simulink model "newsinglecapacitor"  (R2022a)
settings: Solver=VariableStepAuto  StartTime=0.0  StopTime=inf  RelTol=1e-3
undefined symbols (not defined in the file): Ion, Lithium
libraries: spsIdealSwitchLib x9, spsBatteryLib x4, spsCurrentMeasurementLib x1, simulink x1, spsSeriesRLCBranchLib x1, spsVoltageMeasurementLib x1, spspowerguiLib x1
settings Model: Creator=mluser  LastModifiedBy=LENOVO

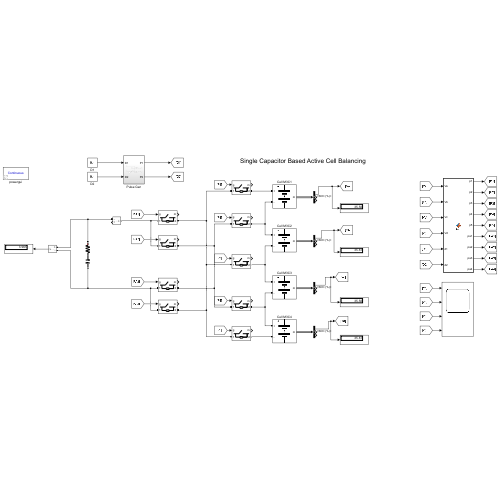
[thumbnail: Simulink's stored preview of the top-level diagram]
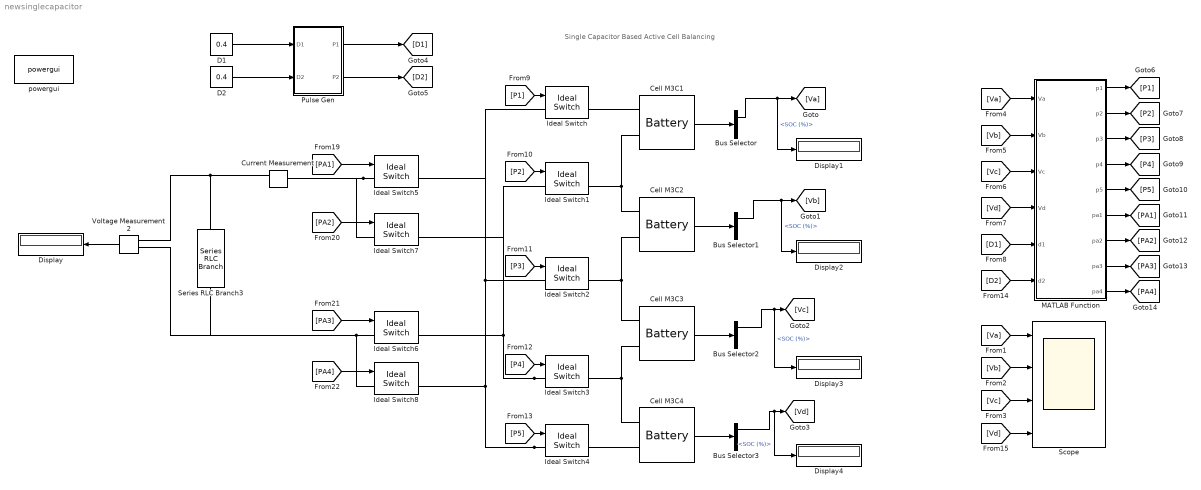
== system newsinglecapacitor ==
  note: Single Capacitor Based Active Cell Balancing
  Bus Selector{,1..3} (4 alike) : BusSelector  OutputSignals=SOC (%),Voltage (V),Current (A)
  Cell M3C1 : spsBatteryLib/Battery  BatType=Lithium-Ion  ShowTempParam=off  ThermalPreset=no  ShowAgeParam=off  NomV=3.7  NomQ=2.6  SOC=35  Batt_Tr=30  PresetModel=off  MaxQ=2.6  MinV=2.775  FullV=4.3068  Dis_rate=1.1304  R=0.014231  Normal_OP=2.3513  expZone="[3.9974      0.12774]"  current=[6.5 13 32.5]  Units=Time  Tci=20  NomT=20  T2=-30  MaxQ2=4.8  FullV2=7.1  Normal_OP2=5.655  expZone2="[6.58           1]"  Rca=0.6  ti=2000  Dp=0  Neq0=0  Tsim=1e6  Ta1=25  Qeol=5.4*0.9  Reol=0.013333*1.2  Char_age=[2.3478, 3]  Dis_age=[2.3478, 10]  N1=1500  N2=10500  N3=1000  N4=1400  Ta2=45  N5=950
  Cell M3C2 : spsBatteryLib/Battery  BatType=Lithium-Ion  ShowTempParam=off  ThermalPreset=no  ShowAgeParam=off  NomV=3.7  NomQ=2.6  SOC=37  Batt_Tr=30  PresetModel=off  MaxQ=2.6  MinV=2.775  FullV=4.3068  Dis_rate=1.1304  R=0.014231  Normal_OP=2.3513  expZone="[3.9974      0.12774]"  current=[6.5 13 32.5]  Units=Time  Tci=20  NomT=20  T2=-30  MaxQ2=4.8  FullV2=7.1  Normal_OP2=5.655  expZone2="[6.58           1]"  Rca=0.6  ti=2000  Dp=0  Neq0=0  Tsim=1e6  Ta1=25  Qeol=5.4*0.9  Reol=0.013333*1.2  Char_age=[2.3478, 3]  Dis_age=[2.3478, 10]  N1=1500  N2=10500  N3=1000  N4=1400  Ta2=45  N5=950
  Cell M3C3 : spsBatteryLib/Battery  BatType=Lithium-Ion  ShowTempParam=off  ThermalPreset=no  ShowAgeParam=off  NomV=3.7  NomQ=2.6  SOC=33  Batt_Tr=30  PresetModel=off  MaxQ=2.6  MinV=2.775  FullV=4.3068  Dis_rate=1.1304  R=0.014231  Normal_OP=2.3513  expZone="[3.9974      0.12774]"  current=[6.5 13 32.5]  Units=Time  Tci=20  NomT=20  T2=-30  MaxQ2=4.8  FullV2=7.1  Normal_OP2=5.655  expZone2="[6.58           1]"  Rca=0.6  ti=2000  Dp=0  Neq0=0  Tsim=1e6  Ta1=25  Qeol=5.4*0.9  Reol=0.013333*1.2  Char_age=[2.3478, 3]  Dis_age=[2.3478, 10]  N1=1500  N2=10500  N3=1000  N4=1400  Ta2=45  N5=950
  Cell M3C4 : spsBatteryLib/Battery  BatType=Lithium-Ion  ShowTempParam=off  ThermalPreset=no  ShowAgeParam=off  NomV=3.7  NomQ=2.6  SOC=38  Batt_Tr=30  PresetModel=off  MaxQ=2.6  MinV=2.775  FullV=4.3068  Dis_rate=1.1304  R=0.014231  Normal_OP=2.3513  expZone="[3.9974      0.12774]"  current=[6.5 13 32.5]  Units=Time  Tci=20  NomT=20  T2=-30  MaxQ2=4.8  FullV2=7.1  Normal_OP2=5.655  expZone2="[6.58           1]"  Rca=0.6  ti=2000  Dp=0  Neq0=0  Tsim=1e6  Ta1=25  Qeol=5.4*0.9  Reol=0.013333*1.2  Char_age=[2.3478, 3]  Dis_age=[2.3478, 10]  N1=1500  N2=10500  N3=1000  N4=1400  Ta2=45  N5=950
  Current Measurement : spsCurrentMeasurementLib/Current Measurement  PhasorSimulation=off  OutputType=Complex  PSBequivalent=0
  D1 : Constant  Value=0.4  SampleTime=1
  D2 : Constant  Value=0.4  SampleTime=1
  Display{,1..4} (5 alike) : Display
  Ideal Switch{,1..8} (9 alike) : spsIdealSwitchLib/Ideal Switch  Ron=0.00001  Lon=0  IC=0  Rs=1e5  Cs=inf  Measurements=on
  MATLAB Function : MATLAB Function  TreatAsAtomicUnit=on
  Pulse Gen : Subsystem
  Scope : Scope  NumInputPorts=4
  Series RLC Branch3 : spsSeriesRLCBranchLib/Series RLC Branch  LConnTagsString=__new0  RConnTagsString=__new0  BranchType=RC  Resistance=0.00001  Inductance=1e-3  SetiL0=off  InitialCurrent=0  Capacitance=1  Setx0=off  InitialVoltage=0  Measurements=None
  Voltage Measurement2 : spsVoltageMeasurementLib/Voltage Measurement  PhasorSimulation=off  OutputType=Complex  PSBequivalent=0
  powergui : spspowerguiLib/powergui  Priority=1  SimulationMode=Continuous  SampleTime=50e-6  frequency=60  Iterations=50  frequencyindice=0  Pbase=100e6  ErrMax=1e-4  UnitsV=kV  UnitsW=MW  buscounter=0  FunctionMessages=off  echomessages=off  EnableUseOfTLC=off  CurrentSourceSwitches=off  DisableSnubberDevices=off  DisableRonSwitches=off  DisableVfSwitches=off  DisplayEquations=off  AutomaticDiscreteSolvers=off  SolverType=Tustin/Backward Euler (TBE)  Interpol=off  ExternalGateDelay=off  methode=off  Ts=100  x0status=blocks  SPID=on  SwTol=0  HookPort=off  NonlinearTolerance=1e-4  nMaxIteration=100  ContinueOnMaxIteration=off  RestoreLinks=warning  ResistiveCurrentMeasurement=off  Frange=[0:2:500]  Ylog=off  Xlog=on  ShowGrid=off  save=off  variable=ZData  structure=0  ZoomFFT=off  StartTime=0.0  cycles=1  DisplayStyle=1  fundamental=60  FreqAxis=off  MaxFrequency=1000  frequencyindicesteady=1  RmsSteady=1  display=off
  wires:
  Pulse Gen/1(P1) -> [D1]
  [PA2] -> Ideal Switch7/1
  Cell M3C3/1 -> Bus Selector2/1
  Bus Selector2/1 -> Display3/1, [Vc]  "<SOC (%)>"
  [PA3] -> Ideal Switch6/1
  D1/1 -> Pulse Gen/1(D1)
  [Va] -> MATLAB Function/1(Va)
  MATLAB Function/3(p3) -> [P3]
  [Vd] -> MATLAB Function/4(Vd)
  [P5] -> Ideal Switch4/1
  MATLAB Function/6(pa1) -> [PA1]
  [PA4] -> Ideal Switch8/1
  Cell M3C1/1 -> Bus Selector/1
  MATLAB Function/4(p4) -> [P4]
  [P4] -> Ideal Switch3/1
  MATLAB Function/8(pa3) -> [PA3]
  [P3] -> Ideal Switch2/1
  [Vb] -> MATLAB Function/2(Vb)
  Bus Selector1/1 -> Display2/1, [Vb]  "<SOC (%)>"
  [P1] -> Ideal Switch/1
  Bus Selector3/1 -> Display4/1, [Vd]  "<SOC (%)>"
  MATLAB Function/5(p5) -> [P5]
  MATLAB Function/1(p1) -> [P1]
  [Vc] -> MATLAB Function/3(Vc)
  Cell M3C2/1 -> Bus Selector1/1
  Pulse Gen/2(P2) -> [D2]
  MATLAB Function/7(pa2) -> [PA2]
  [D2] -> MATLAB Function/6(d2)
  [PA1] -> Ideal Switch5/1
  [P2] -> Ideal Switch1/1
  MATLAB Function/2(p2) -> [P2]
  Cell M3C4/1 -> Bus Selector3/1
  MATLAB Function/9(pa4) -> [PA4]
  D2/1 -> Pulse Gen/2(D2)
  Bus Selector/1 -> Display1/1, [Va]  "<SOC (%)>"
  Voltage Measurement2/1 -> Display/1
  [D1] -> MATLAB Function/5(d1)
  [Va] -> Scope/1
  [Vb] -> Scope/2
  [Vc] -> Scope/3
  [Vd] -> Scope/4
  connections:
  Cell M3C4/LConn2 -- Ideal Switch4/RConn1
  Ideal Switch8/LConn1 -- Voltage Measurement2/LConn2 -- Series RLC Branch3/RConn1 -- Ideal Switch6/LConn1
  Series RLC Branch3/LConn1 -- Voltage Measurement2/LConn1 -- Current Measurement/RConn1
  Ideal Switch3/RConn1 -- Cell M3C3/LConn2 -- Cell M3C4/LConn1
  Ideal Switch3/LConn1 -- Ideal Switch6/RConn1 -- Ideal Switch7/RConn1 -- Ideal Switch1/LConn1
  Ideal Switch2/RConn1 -- Cell M3C2/LConn2 -- Cell M3C3/LConn1
  Ideal Switch1/RConn1 -- Cell M3C1/LConn2 -- Cell M3C2/LConn1
  Ideal Switch4/LConn1 -- Ideal Switch5/RConn1 -- Ideal Switch/LConn1 -- Ideal Switch2/LConn1 -- Ideal Switch8/RConn1
  Ideal Switch5/LConn1 -- Current Measurement/LConn1 -- Ideal Switch7/LConn1
  Cell M3C1/LConn1 -- Ideal Switch/RConn1

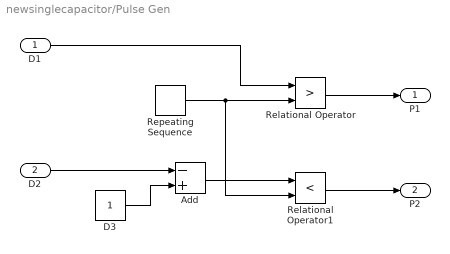
== system newsinglecapacitor/Pulse Gen ==
  D1 : Inport
  D2 : Inport  Port=2
  Add : Sum  Inputs=-+
  D3 : Constant
  Relational Operator : RelationalOperator  Operator=>  OutDataTypeStr=boolean  RndMeth=Simplest  InputSameDT=off
  Relational Operator1 : RelationalOperator  Operator=<  OutDataTypeStr=boolean  RndMeth=Simplest  InputSameDT=off
  Repeating Sequence : simulink/Sources/Repeating Sequence  rep_seq_t=[0 0.5/10 1/10]  rep_seq_y=[0 1 0]
  P1 : Outport  VectorParamsAs1DForOutWhenUnconnected=off
  P2 : Outport  Port=2  VectorParamsAs1DForOutWhenUnconnected=off
  wires:
  Add/1 -> Relational Operator1/1
  D3/1 -> Add/2
  D2/1 -> Add/1
  Relational Operator1/1 -> P2/1
  Relational Operator/1 -> P1/1
  D1/1 -> Relational Operator/1
  Repeating Sequence/1 -> Relational Operator/2, Relational Operator1/2

== matlab function newsinglecapacitor/MATLAB Function ==
  data: Va input; p1 output; Vb input; Vc input; Vd input; p2 output; p3 output; p4 output; p5 output; pa1 output; pa2 output; pa3 output; pa4 output; d1 input; d2 input
function [p1,p2,p3,p4,p5,pa1,pa2,pa3,pa4] = fcn(Va,Vb,Vc,Vd,d1,d2)

[~,high]=max([Va,Vb,Vc,Vd]);
[~,low]=min([Va,Vb,Vc,Vd]);

if d1==1
    switch high
    
        case 1    
            p1=1;
            p2=1;
            p3=0;
            p4=0;
            p5=0;

            pa1=1;
            pa2=0;

            pa3=1;
            pa4=0;

        case 2    
            p1=0;
            p2=1;
            p3=1;
            p4=0;
            p5=0;

            pa1=0;
            pa2=1;

            pa3=0;
            pa4=1;

        case 3    
            p1=0;
            p2=0;
            p3=1;
            p4=1;
            p5=0;

            pa1=1;
            pa2=0;

            pa3=1;
            pa4=0;

         case 4    
            p1=0;
            p2=0;
            p3=0;
            p4=1;
            p5=1;

            pa1=0;
            pa2=1;

            pa3=0;
            pa4=1;

        otherwise            

            p1=0;
            p2=0;
            p3=0;
            p4=0;
            p5=0;

            pa1=0;
            pa2=0;

            pa3=0;
            pa4=0;

            
    end
    
elseif d2==1    

    switch low
    
        case 1    
            p1=1;
            p2=1;
            p3=0;
            p4=0;
            p5=0;

            pa1=1;
            pa2=0;

            pa3=1;
            pa4=0;

        case 2    
            p1=0;
            p2=1;
            p3=1;
            p4=0;
            p5=0;

            pa1=0;
            pa2=1;

            pa3=0;
            pa4=1;

        case 3    
            p1=0;
            p2=0;
            p3=1;
            p4=1;
            p5=0;

            pa1=1;
            pa2=0;

            pa3=1;
            pa4=0;

         case 4    
            p1=0;
            p2=0;
            p3=0;
            p4=1;
            p5=1;

            pa1=0;
            pa2=1;

            pa3=0;
            pa4=1;
            
       otherwise            

            p1=0;
            p2=0;
            p3=0;
            p4=0;
            p5=0;

            pa1=0;
            pa2=0;

            pa3=0;
            pa4=0;
            

    end
    
else
            p1=0;
            p2=0;
            p3=0;
            p4=0;
            p5=0;

            pa1=0;
            pa2=0;

            pa3=0;
            pa4=0;
    
    
end


end
